simulink model "Trajectory_Generator"  (R2017b)
settings: Solver=VariableStepAuto  StartTime=0.0  StopTime=10.0  RelTol=1e-3
settings Model: Creator=Kalana  LastModifiedBy=Kalana

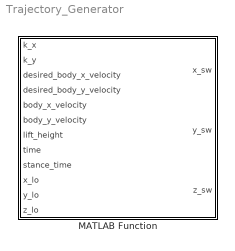
== system Trajectory_Generator ==
  MATLAB Function : MATLAB Function  TreatAsAtomicUnit=on

== matlab function Trajectory_Generator/MATLAB Function ==
  data: k_x input; x_sw output; k_y input; desired_body_x_velocity input; desired_body_y_velocity input; body_x_velocity input; body_y_velocity input; lift_height input; time input; stance_time input; x_lo input; y_lo input; z_lo input; y_sw output; z_sw output
function [x_sw, y_sw, z_sw] = Trajectory_Generator(k_x, k_y, desired_body_x_velocity, desired_body_y_velocity, body_x_velocity, body_y_velocity, lift_height, time, stance_time, x_lo, y_lo, z_lo)

yf = ((0.5*body_y_velocity*stance_time) - (k_y*(desired_body_y_velocity - body_y_velocity)));
xf = ((0.5*body_x_velocity*stance_time) - (k_x*(desired_body_x_velocity - body_x_velocity)));

phi = (2*3.14*time)/stance_time;

x_sw = (x_lo + ((xf - x_lo)*(phi - sin(phi))/(2*3.14)));
y_sw = (y_lo + ((yf - y_lo)*(phi - sin(phi))/(2*3.14)));
z_sw = (z_lo + (lift_height*(1 - cos(phi))/2));
